simulink model "EXPERIMENT_04_B"  (R2023b)
settings: Solver=VariableStepAuto  StartTime=0.0  StopTime=10.0  RelTol=1e-3
undefined symbols (not defined in the file): Angle, Magnitude
libraries: spsCurrentMeasurementLib x3, spsVoltageMeasurementLib x3, spsSeriesRLCBranchLib x2, spsLinearTransformerLib x2, spsACVoltageSourceLib x1, sps_lib x1
settings Model: Creator=deves  LastModifiedBy=deves

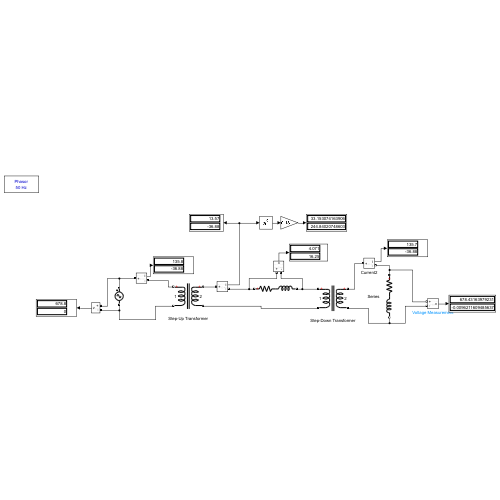
[thumbnail: Simulink's stored preview of the top-level diagram]
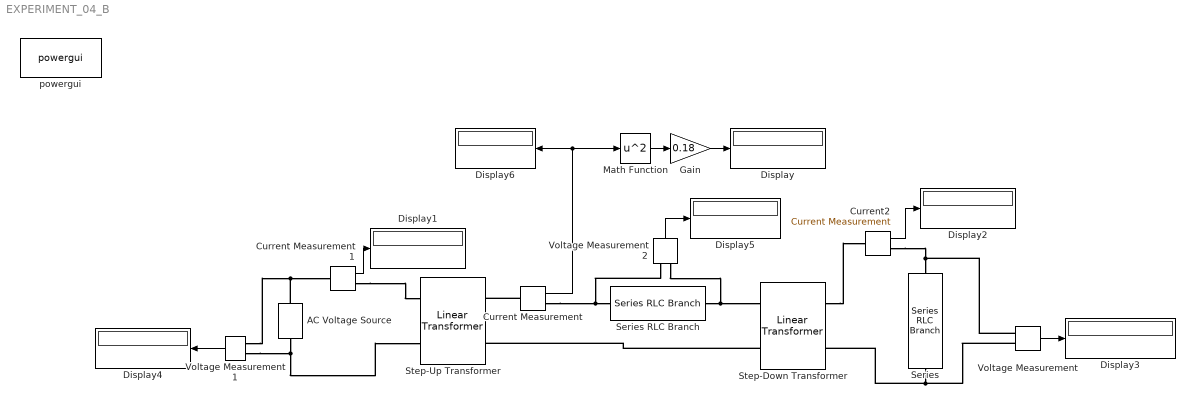
== system EXPERIMENT_04_B ==
  AC Voltage Source : spsACVoltageSourceLib/AC Voltage Source  Amplitude=480*sqrt(2)  Phase=0  Frequency=50  SampleTime=0  Measurements=None  BusType=swing  Pref=10e3  Qref=0  Qmin=-inf  Qmax=+inf
  Current Measurement : spsCurrentMeasurementLib/Current Measurement  PhasorSimulation=on  OutputType=Magnitude-Angle  PSBequivalent=0
  Current Measurement1 : spsCurrentMeasurementLib/Current Measurement  PhasorSimulation=on  OutputType=Magnitude-Angle  PSBequivalent=0
  Current2 : spsCurrentMeasurementLib/Current Measurement  PhasorSimulation=on  OutputType=Magnitude-Angle  PSBequivalent=0
  Display{,1..6} (7 alike) : Display
  Gain : Gain  Gain=0.18
  Math Function : Math  Operator=square
  Series : spsSeriesRLCBranchLib/Series RLC Branch  LConnTagsString=__new0  RConnTagsString=__new0  BranchType=RL  Resistance=4  Inductance=3/(2*pi*50)  SetiL0=off  InitialCurrent=0  Capacitance=0  Setx0=off  InitialVoltage=0  Measurements=None
  Series RLC Branch : spsSeriesRLCBranchLib/Series RLC Branch  LConnTagsString=__new0  RConnTagsString=__new0  BranchType=RL  Resistance=0.18  Inductance=0.24/(2*pi*50)  SetiL0=off  InitialCurrent=0  Capacitance=0  Setx0=off  InitialVoltage=0  Measurements=None
  Step-Down Transformer : spsLinearTransformerLib/Linear Transformer  UNITS=SI  NominalPower=[ 10000 50 ]  winding1=[4800 0 0]  winding2=[480 0 0]  ThreeWindings=off  winding3=[3.15e+05 29234 3722.2]  RmLm=[3.394e+06 10804]  Measurements=None  DataType=on
  Step-Up Transformer : spsLinearTransformerLib/Linear Transformer  UNITS=pu  NominalPower=[10000 50 ]  winding1=[480 0 0]  winding2=[4800 0 0]  ThreeWindings=off  winding3=[3.15e+05 0.0014142 0.056568]  RmLm=[707.08 707.12]  Measurements=None  DataType=off
  Voltage Measurement : spsVoltageMeasurementLib/Voltage Measurement  PhasorSimulation=on  OutputType=Magnitude-Angle  PSBequivalent=0
  Voltage Measurement1 : spsVoltageMeasurementLib/Voltage Measurement  PhasorSimulation=on  OutputType=Magnitude-Angle  PSBequivalent=0
  Voltage Measurement2 : spsVoltageMeasurementLib/Voltage Measurement  PhasorSimulation=on  OutputType=Magnitude-Angle  PSBequivalent=0
  powergui : sps_lib/powergui  Priority=1  SimulationMode=Phasor  SampleTime=50e-6  frequency=50  Iterations=50  frequencyindice=50  Pbase=100e6  ErrMax=1e-4  UnitsV=kV  UnitsW=MW  buscounter=0  FunctionMessages=off  echomessages=off  EnableUseOfTLC=off  CurrentSourceSwitches=off  DisableSnubberDevices=off  DisableRonSwitches=off  DisableVfSwitches=off  DisplayEquations=off  AutomaticDiscreteSolvers=off  SolverType=Tustin/Backward Euler (TBE)  Interpol=off  ExternalGateDelay=off  methode=off  Ts=100  x0status=blocks  SPID=on  SwTol=0  HookPort=off  NonlinearTolerance=1e-4  nMaxIteration=100  ContinueOnMaxIteration=off  RestoreLinks=warning  ResistiveCurrentMeasurement=off  Frange=[0:2:500]  Ylog=off  Xlog=on  ShowGrid=off  save=off  variable=ZData  structure=0  ZoomFFT=off  StartTime=0.0  cycles=1  DisplayStyle=1  fundamental=60  FreqAxis=off  MaxFrequency=1000  frequencyindicesteady=1  RmsSteady=1  display=off
  wires:
  Current Measurement/1 -> Math Function/1, Display6/1
  Gain/1 -> Display/1
  Math Function/1 -> Gain/1
  Current Measurement1/1 -> Display1/1
  Current2/1 -> Display2/1
  Voltage Measurement2/1 -> Display5/1
  Voltage Measurement/1 -> Display3/1
  Voltage Measurement1/1 -> Display4/1
  connections:
  AC Voltage Source/LConn1 -- Step-Up Transformer/LConn2 -- Voltage Measurement1/LConn2
  Series RLC Branch/RConn1 -- Step-Down Transformer/LConn1 -- Voltage Measurement2/LConn2
  Step-Down Transformer/LConn2 -- Step-Up Transformer/RConn2
  Series/RConn1 -- Voltage Measurement/LConn2 -- Step-Down Transformer/RConn2
  Current Measurement/LConn1 -- Step-Up Transformer/RConn1
  Current Measurement/RConn1 -- Voltage Measurement2/LConn1 -- Series RLC Branch/LConn1
  AC Voltage Source/RConn1 -- Voltage Measurement1/LConn1 -- Current Measurement1/LConn1
  Current Measurement1/RConn1 -- Step-Up Transformer/LConn1
  Step-Down Transformer/RConn1 -- Current2/LConn1
  Current2/RConn1 -- Voltage Measurement/LConn1 -- Series/LConn1
